simulink model "SPWM_2closed_loop"  (R2022b)
settings: Solver=FixedStepDiscrete  StartTime=0.0  StopTime=0.2  FixedStep=1e-6  RelTol=1e-3
InitFcn:
  | f = 10e3;
  | Ts = 1/f;
  | Vdc = 850;
  | L1 = 0.9e-3;
  | C = 40e-6;
  | R = 0.1;
  | L2 = 0.1e-3;
  | RC = 0.01;
undefined symbols (not defined in the file): Simulation
libraries: spsSeriesRLCBranchLib x11, spsMosfetLib x6, spsThreePhaseVIMeasurementLib x4, spsGroundLib x2, simulink x1, spsThreePhaseSourceLib x1, spsDCVoltageSourceLib x1, spsMultimeterLib x1, sps_lib x1
settings Model: Creator=Li  LastModifiedBy=Li
settings DataIOCC: ReturnWorkspaceOutputs=off

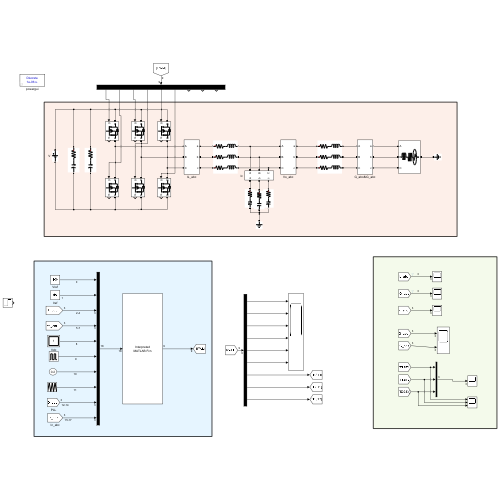
[thumbnail: Simulink's stored preview of the top-level diagram]
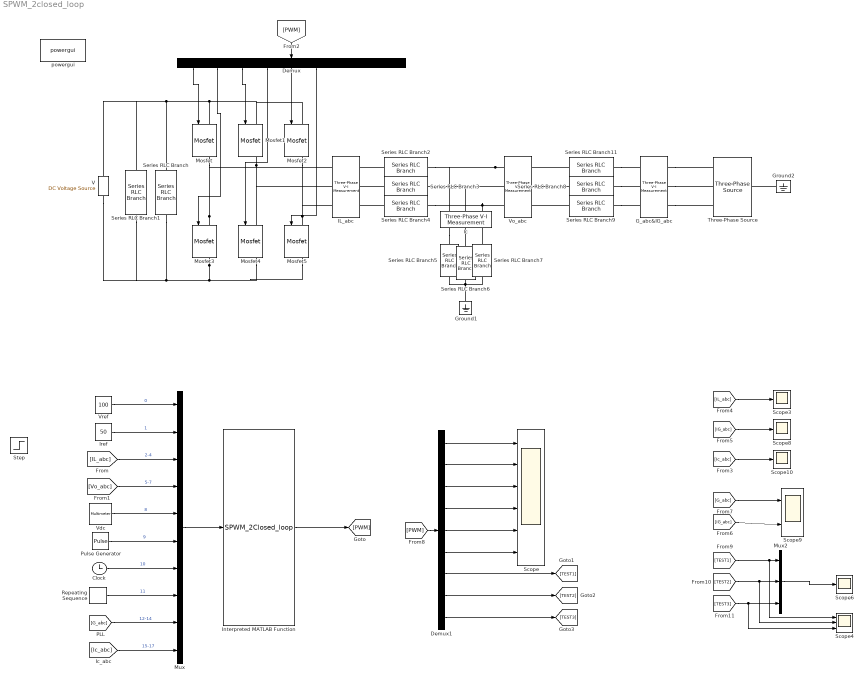
== system SPWM_2closed_loop ==
  Clock : Clock
  Demux : Demux  Outputs=9
  Demux1 : Demux  Outputs=9
  G_abc&IG_abc : spsThreePhaseVIMeasurementLib/Three-Phase V-I Measurement  VoltageMeasurement=phase-to-ground  SetLabelV=on  LabelV=G_abc  Vpu=off  VpuLL=off  CurrentMeasurement=yes  SetLabelI=on  LabelI=IG_abc  Ipu=off  Pbase=100e6  Vbase=500e3  OutputType=Complex  PhasorSimulation=off  PSBequivalent=0
  Ground1 : spsGroundLib/Ground  LConnTagsString=a
  Ground2 : spsGroundLib/Ground  LConnTagsString=a
  IL_abc : spsThreePhaseVIMeasurementLib/Three-Phase V-I Measurement  VoltageMeasurement=no  SetLabelV=on  LabelV=Vabc  Vpu=off  VpuLL=off  CurrentMeasurement=yes  SetLabelI=on  LabelI=IL_abc  Ipu=off  Pbase=100e6  Vbase=500e3  OutputType=Complex  PhasorSimulation=off  PSBequivalent=0
  Ic : spsThreePhaseVIMeasurementLib/Three-Phase V-I Measurement  VoltageMeasurement=no  SetLabelV=on  LabelV=Vabc  Vpu=off  VpuLL=off  CurrentMeasurement=yes  SetLabelI=on  LabelI=Ic_abc  Ipu=off  Pbase=100e6  Vbase=500e3  OutputType=Complex  PhasorSimulation=off  PSBequivalent=0
  Interpreted MATLAB Function : MATLABFcn  MATLABFcn=SPWM_2Closed_loop  OutputDimensions=9
  Iref : Constant  Value=50
  Mosfet{,1..5} (6 alike) : spsMosfetLib/Mosfet  Ron=0.1  Lon=0  Rd=0.01  Vfd=0  IC=0  Rs=1e5  Cs=inf  Measurements=on
  Mux : Mux  Inputs=10
  Mux2 : Mux  Inputs=3
  Pulse Generator : DiscretePulseGenerator  PulseType=Time based  Period=Ts  PulseWidth=50
  Repeating Sequence : simulink/Sources/Repeating Sequence  rep_seq_t=[0 Ts/2 Ts]  rep_seq_y=[0 1 0]
  Scope : Scope  NumInputPorts=6
  Scope{3,6,8,10} (4 alike) : Scope
  Scope4 : Scope  NumInputPorts=3
  Scope9 : Scope  NumInputPorts=2
  Series RLC Branch : spsSeriesRLCBranchLib/Series RLC Branch  LConnTagsString=__new0  RConnTagsString=__new0  BranchType=RC  Resistance=1e-9  Inductance=1e-3  SetiL0=off  InitialCurrent=0  Capacitance=660e-6  Setx0=off  InitialVoltage=0  Measurements=None
  Series RLC Branch1 : spsSeriesRLCBranchLib/Series RLC Branch  LConnTagsString=__new0  RConnTagsString=__new0  BranchType=RC  Resistance=1e-9  Inductance=1e-3  SetiL0=off  InitialCurrent=0  Capacitance=23.5e-6  Setx0=off  InitialVoltage=0  Measurements=None
  Series RLC Branch11 : spsSeriesRLCBranchLib/Series RLC Branch  LConnTagsString=__new0  RConnTagsString=__new0  BranchType=RL  Resistance=R  Inductance=L2  SetiL0=off  InitialCurrent=0  Capacitance=1e-3  Setx0=off  InitialVoltage=0  Measurements=None
  Series RLC Branch2 : spsSeriesRLCBranchLib/Series RLC Branch  LConnTagsString=__new0  RConnTagsString=__new0  BranchType=RL  Resistance=R  Inductance=L1  SetiL0=off  InitialCurrent=0  Capacitance=1e-3  Setx0=off  InitialVoltage=0  Measurements=None
  Series RLC Branch3 : spsSeriesRLCBranchLib/Series RLC Branch  LConnTagsString=__new0  RConnTagsString=__new0  BranchType=RL  Resistance=R  Inductance=L1  SetiL0=off  InitialCurrent=0  Capacitance=1e-3  Setx0=off  InitialVoltage=0  Measurements=None
  Series RLC Branch4 : spsSeriesRLCBranchLib/Series RLC Branch  LConnTagsString=__new0  RConnTagsString=__new0  BranchType=RL  Resistance=R  Inductance=L1  SetiL0=off  InitialCurrent=0  Capacitance=1e-3  Setx0=off  InitialVoltage=0  Measurements=None
  Series RLC Branch5 : spsSeriesRLCBranchLib/Series RLC Branch  LConnTagsString=__new0  RConnTagsString=__new0  BranchType=RC  Resistance=RC  Inductance=Simulation.Inverter.Params.L1  SetiL0=off  InitialCurrent=0  Capacitance=C  Setx0=off  InitialVoltage=0  Measurements=None
  Series RLC Branch6 : spsSeriesRLCBranchLib/Series RLC Branch  LConnTagsString=__new0  RConnTagsString=__new0  BranchType=RC  Resistance=RC  Inductance=Simulation.Inverter.Params.L1  SetiL0=off  InitialCurrent=0  Capacitance=C  Setx0=off  InitialVoltage=0  Measurements=None
  Series RLC Branch7 : spsSeriesRLCBranchLib/Series RLC Branch  LConnTagsString=__new0  RConnTagsString=__new0  BranchType=RC  Resistance=RC  Inductance=Simulation.Inverter.Params.L1  SetiL0=off  InitialCurrent=0  Capacitance=C  Setx0=off  InitialVoltage=0  Measurements=None
  Series RLC Branch8 : spsSeriesRLCBranchLib/Series RLC Branch  LConnTagsString=__new0  RConnTagsString=__new0  BranchType=RL  Resistance=R  Inductance=L2  SetiL0=off  InitialCurrent=0  Capacitance=1e-3  Setx0=off  InitialVoltage=0  Measurements=None
  Series RLC Branch9 : spsSeriesRLCBranchLib/Series RLC Branch  LConnTagsString=__new0  RConnTagsString=__new0  BranchType=RL  Resistance=R  Inductance=L2  SetiL0=off  InitialCurrent=0  Capacitance=1e-3  Setx0=off  InitialVoltage=0  Measurements=None
  Step : Step  Time=0.1  Before=100  After=150  SampleTime=0
  Three-Phase Source : spsThreePhaseSourceLib/Three-Phase Source  InternalConnection=Yn  VoltagePhases=off  Voltage=380  PhaseAngle=0  Voltage_phases=[25e3 25e3 25e3]/sqrt(3)  PhaseAngles_phases=[0 -120 +120]  Frequency=50  NonIdealSource=on  SpecifyImpedance=off  Resistance=1e-6  Inductance=1e-6  ShortCircuitLevel=100e6  BaseVoltage=380  XRratio=7  BusType=swing  Pref=10e3  Qref=0  Prefabc=[10e3, 10e3, 10e3]  Qrefabc=[0, 0, 0]  Qmin=-inf  Qmax=inf
  V : spsDCVoltageSourceLib/DC Voltage Source  Amplitude=Vdc  Measurements=Voltage
  Vdc : spsMultimeterLib/Multimeter  L=1  sel=1  yselected={}  Gain=1  OutputType=Complex  PlotAtSimulationStop=off  PhasorSimulation=off
  Vo_abc : spsThreePhaseVIMeasurementLib/Three-Phase V-I Measurement  VoltageMeasurement=phase-to-ground  SetLabelV=on  LabelV=Vo_abc  Vpu=off  VpuLL=off  CurrentMeasurement=no  SetLabelI=on  LabelI=Iabc  Ipu=off  Pbase=100e6  Vbase=500e3  OutputType=Complex  PhasorSimulation=off  PSBequivalent=0
  Vref : Constant  Value=100
  powergui : sps_lib/powergui  Priority=1  SimulationMode=Discrete  SampleTime=1e-6  frequency=60  Iterations=50  frequencyindice=0  Pbase=100e6  ErrMax=1e-4  UnitsV=kV  UnitsW=MW  buscounter=0  FunctionMessages=off  echomessages=off  EnableUseOfTLC=off  CurrentSourceSwitches=off  DisableSnubberDevices=off  DisableRonSwitches=off  DisableVfSwitches=off  DisplayEquations=off  AutomaticDiscreteSolvers=off  SolverType=Tustin/Backward Euler (TBE)  Interpol=off  ExternalGateDelay=off  methode=off  Ts=100  x0status=blocks  SPID=on  SwTol=0  HookPort=off  NonlinearTolerance=1e-4  nMaxIteration=100  ContinueOnMaxIteration=off  RestoreLinks=warning  ResistiveCurrentMeasurement=off  Frange=[0:2:500]  Ylog=off  Xlog=on  ShowGrid=off  save=off  variable=ZData  structure=0  ZoomFFT=off  StartTime=0.0  cycles=1  DisplayStyle=1  fundamental=60  FreqAxis=off  MaxFrequency=1000  frequencyindicesteady=1  RmsSteady=1  display=off
  wires:
  Vref/1 -> Mux/1  "0"
  [IL_abc] -> Mux/3  "2-4"
  Vdc/1 -> Mux/5  "8"
  Mux/1 -> Interpreted MATLAB Function/1
  Interpreted MATLAB Function/1 -> [PWM]
  Pulse Generator/1 -> Mux/6  "9"
  Clock/1 -> Mux/7  "10"
  Repeating Sequence/1 -> Mux/8  "11"
  [PWM] -> Demux/1
  Demux/1 -> Mosfet/1
  Demux/2 -> Mosfet3/1
  Demux/3 -> Mosfet1/1
  Demux/4 -> Mosfet4/1
  Demux/5 -> Mosfet2/1
  Demux/6 -> Mosfet5/1
  Demux1/1 -> Scope/1
  Demux1/2 -> Scope/2
  Demux1/3 -> Scope/3
  Demux1/4 -> Scope/4
  Demux1/5 -> Scope/5
  Demux1/6 -> Scope/6
  Demux1/7 -> [TEST1]
  Demux1/9 -> [TEST3]
  Mux2/1 -> Scope6/1
  [Vo_abc] -> Mux/4  "5-7"
  [G_abc] -> Mux/9  "12-14"
  [IL_abc] -> Scope3/1
  [IG_abc] -> Scope8/1
  [G_abc] -> Scope9/1
  [IG_abc] -> Scope9/2
  [Ic_abc] -> Mux/10  "15-17"
  [Ic_abc] -> Scope10/1
  [PWM] -> Demux1/1
  Demux1/8 -> [TEST2]
  [TEST1] -> Scope4/1, Mux2/1
  [TEST2] -> Scope4/2, Mux2/2
  [TEST3] -> Scope4/3, Mux2/3
  Iref/1 -> Mux/2  "1"
  connections:
  Series RLC Branch5/RConn1 -- Series RLC Branch7/RConn1 -- Series RLC Branch6/RConn1 -- Ground1/LConn1
  Ic/LConn2 -- Series RLC Branch3/RConn1 -- Vo_abc/LConn2
  Series RLC Branch/LConn1 -- V/RConn1 -- Series RLC Branch1/LConn1 -- Mosfet2/LConn1 -- Mosfet1/LConn1 -- Mosfet/LConn1
  Mosfet1/RConn1 -- Mosfet4/LConn1 -- IL_abc/LConn2
  Mosfet3/LConn1 -- Mosfet/RConn1 -- IL_abc/LConn1
  Ic/LConn3 -- Series RLC Branch4/RConn1 -- Vo_abc/LConn3
  Mosfet5/LConn1 -- Mosfet2/RConn1 -- IL_abc/LConn3
  Mosfet3/RConn1 -- V/LConn1 -- Series RLC Branch1/RConn1 -- Series RLC Branch/RConn1 -- Mosfet5/RConn1 -- Mosfet4/RConn1
  Series RLC Branch8/LConn1 -- Vo_abc/RConn2
  Series RLC Branch9/LConn1 -- Vo_abc/RConn3
  Series RLC Branch11/LConn1 -- Vo_abc/RConn1
  Ground2/LConn1 -- Three-Phase Source/LConn1
  Series RLC Branch11/RConn1 -- G_abc&IG_abc/LConn1
  Series RLC Branch8/RConn1 -- G_abc&IG_abc/LConn2
  Series RLC Branch9/RConn1 -- G_abc&IG_abc/LConn3
  G_abc&IG_abc/RConn1 -- Three-Phase Source/RConn1
  G_abc&IG_abc/RConn2 -- Three-Phase Source/RConn2
  G_abc&IG_abc/RConn3 -- Three-Phase Source/RConn3
  Ic/RConn1 -- Series RLC Branch5/LConn1
  Series RLC Branch6/LConn1 -- Ic/RConn2
  Series RLC Branch7/LConn1 -- Ic/RConn3
  Series RLC Branch2/LConn1 -- IL_abc/RConn1
  Series RLC Branch3/LConn1 -- IL_abc/RConn2
  Series RLC Branch4/LConn1 -- IL_abc/RConn3
  Vo_abc/LConn1 -- Series RLC Branch2/RConn1 -- Ic/LConn1
